simulink model "modulador_torque_en_planta"  (R2023b)
settings: Solver=VariableStepAuto  StartTime=0.0  StopTime=10  RelTol=1e-3
settings Model: Creator=nicol  LastModifiedBy=nicol

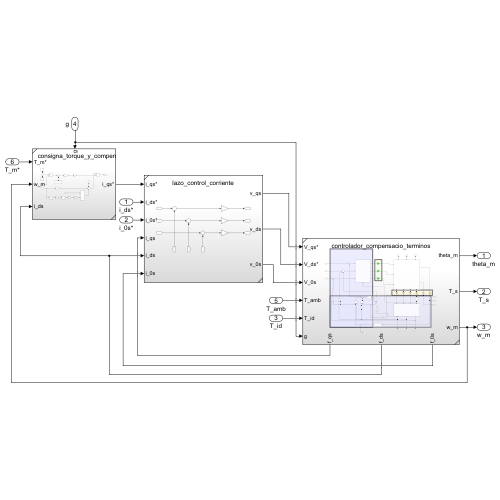
[thumbnail: Simulink's stored preview of the top-level diagram]
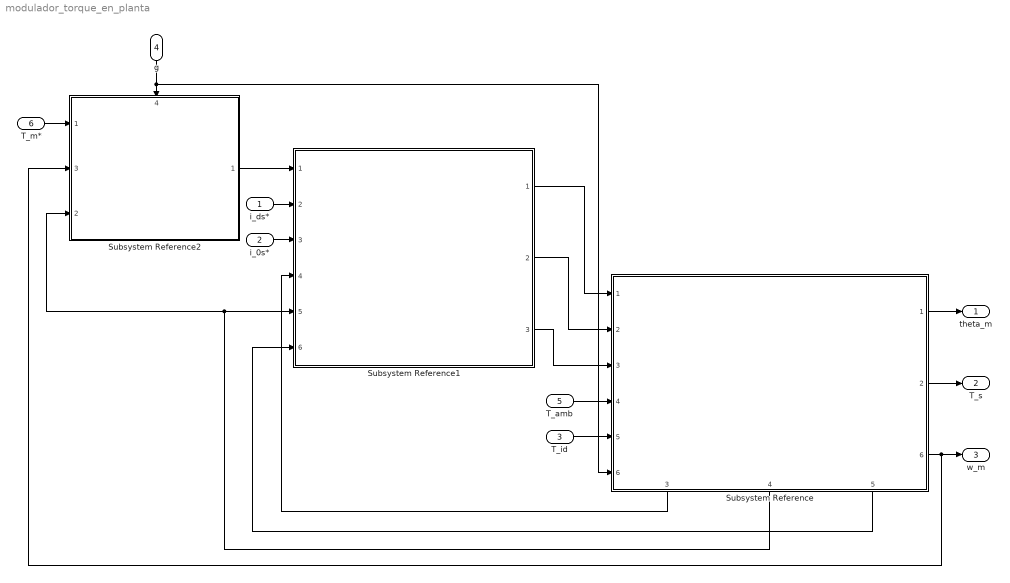
== system modulador_torque_en_planta ==
  i_ds* : Inport
  i_0s* : Inport  Port=2
  T_id : Inport  Port=3
  g : Inport  Port=4
  T_amb : Inport  Port=5
  T_m* : Inport  Port=6
  Subsystem Reference : Subsystem  ReferencedSubsystem=controlador_compensacio_terminos
      settings: PortSchema="{\"entries\":[{\"content\":{\"sides\":[{\"content\":{\"connectorIds\":[\"In1\",\"In2\",\"In3\",\"In4\",\"In5\",\"In6\"]},\"type\":\"ConnectorPlacement.EquallySpacedRectSide\",\"uuid\":\"b1c276fb-f5d1-4d19-a6ea-7d1a09b8349f\"},{\"content\":{\"connectorIds\":[\"Out1\",\"Out2\",\"Out6\"],\"side\":\"RIGHT\"},\"type\":\"ConnectorPlacement.EquallySpacedRectSide\",\"uuid\":\"27d8bc07-3c44-4620-a597-2ff8ea4c23ab\"},{\"content\":{\"side\":\"TOP\"},\"type\":\"ConnectorPlacement.EquallySpacedRectSide\",\"uuid\":\"3df4da6c-73e7-44ec-b643-950781e1e40a\"},{\"content\":{\"connectorIds\":[\"Out3\",\"Out4\",\"Out5\"],\"side\":\"BOTTOM\"},\"type\":\"ConnectorPlacement.EquallySpacedRectSide\",\"uuid\":\"41447b30-fc5c-45b8-8eff-edc74dd03fa8\"}]},\"type\":\"ConnectorPlacement.EquallySpacedConnector\",\"uuid\":\"40e819b3-95dd-49e4-ad1c-9b4691395cc7\"}],\"packageUris\":[\"http://schema.mathworks.com/mf0/Connector/R2020b\"],\"version\":\"1.0\"}"
  Subsystem Reference1 : Subsystem  ReferencedSubsystem=lazo_control_corriente
  Subsystem Reference2 : Subsystem  ReferencedSubsystem=consigna_torque_y_compensaciones
      settings: PortSchema="{\"entries\":[{\"content\":{\"sides\":[{\"content\":{\"connectorIds\":[\"In1\",\"In3\",\"In2\"]},\"type\":\"ConnectorPlacement.EquallySpacedRectSide\",\"uuid\":\"1885e5f5-f6ac-4449-9525-6488a0e1a0df\"},{\"content\":{\"connectorIds\":[\"Out1\"],\"side\":\"RIGHT\"},\"type\":\"ConnectorPlacement.EquallySpacedRectSide\",\"uuid\":\"5c837a64-ddee-40b5-814c-ed51094d23eb\"},{\"content\":{\"connectorIds\":[\"In4\"],\"side\":\"TOP\"},\"type\":\"ConnectorPlacement.EquallySpacedRectSide\",\"uuid\":\"3b41ea9d-e5d3-43cd-ba13-1502040c9f0f\"}]},\"type\":\"ConnectorPlacement.EquallySpacedConnector\",\"uuid\":\"b9cdf7e5-86b7-4e3e-be26-3bae3f56036b\"}],\"packageUris\":[\"http://schema.mathworks.com/mf0/Connector/R2020b\"],\"version\":\"1.0\"}"
  theta_m : Outport
  T_s : Outport  Port=2
  w_m : Outport  Port=3
  wires:
  Subsystem Reference2/1 -> Subsystem Reference1/1
  Subsystem Reference1/1 -> Subsystem Reference/1
  Subsystem Reference1/2 -> Subsystem Reference/2
  Subsystem Reference1/3 -> Subsystem Reference/3
  i_ds*/1 -> Subsystem Reference1/2
  i_0s*/1 -> Subsystem Reference1/3
  Subsystem Reference/3 -> Subsystem Reference1/4
  Subsystem Reference/4 -> Subsystem Reference1/5, Subsystem Reference2/2
  Subsystem Reference/5 -> Subsystem Reference1/6
  T_id/1 -> Subsystem Reference/5
  Subsystem Reference/1 -> theta_m/1
  Subsystem Reference/2 -> T_s/1
  Subsystem Reference/6 -> Subsystem Reference2/3, w_m/1
  g/1 -> Subsystem Reference/6, Subsystem Reference2/4
  T_amb/1 -> Subsystem Reference/4
  T_m*/1 -> Subsystem Reference2/1
